simulink model "ass2_test_additions"  (R2022b)
settings: Solver=FixedStepAuto  StartTime=0.0  StopTime=10.0  FixedStep=1e-3  RelTol=1e-3  EnableMultiTasking=on
undefined symbols (not defined in the file): a, b, c, D0, D1, D10, D11, D12, D13, D2, D3, D4, D5, D6, D7, D8, D9, PTA0, PTA1, PTA2, PTB23, PTB9, PTC16, PTC17, PTC2, PTC3, PTC4, PTD0, PTD1, PTD2, PTD3
libraries: frdmk64flib x18, simulink x2, dspstat3 x1, hdlsllib x1
settings Model: ExtModeTrigDuration=5  Creator=hinda  LastModifiedBy=Venka
settings SolverCC: AlgebraicLoopSolver=TrustRegion
settings OptimizationCC: EnhancedBackFolding=on  PassReuseOutputArgsAs=Individual arguments  ZeroExternalMemoryAtStartup=off  ZeroInternalMemoryAtStartup=off  MaxStackSize=64  OptimizeBlockOrder=speed  DifferentSizesBufferReuse=on  OptimizationCustomize=off  EfficientTunableParamExpr=on
settings DebuggingCC: ParameterTunabilityLossMsg=error  UnconnectedInputMsg=warning  UnconnectedOutputMsg=warning  UnconnectedLineMsg=warning  SFMachineParentedDataDiag=warning
settings HardwareCC: ProdBitPerPointer=32  ProdBitPerSizeT=32  ProdBitPerPtrDiffT=32  ProdLargestAtomicInteger=Long  ProdLargestAtomicFloat=Double  ProdWordSize=32  ProdHWDeviceType=ARM Compatible->ARM Cortex
settings ModelReferenceCC: EnableRefExpFcnMdlSchedulingChecks=on
settings SFSimCC: MATLABDynamicMemAlloc=off
settings RTWCC: Description=Embedded Coder  SystemTargetFile=ert.tlc  HardwareBoard=NXP FRDM-K64F  TLCOptions="-aInlineSetEventsForThisBaseRateFcn=TLC_FALSE -aSuppressMultiTaskScheduler=TLC_FALSE  -aRateBasedStepFcn=0"  TemplateMakefile=ert_default_tmf  Toolchain=GNU Tools for ARM Embedded Processors
settings CodeAppCC: ForceParamTrailComments=on  IgnoreCustomStorageClasses=off  OperatorAnnotations=on  SimulinkDataObjDesc=on  SFDataObjDesc=on  InsertBlockDesc=on

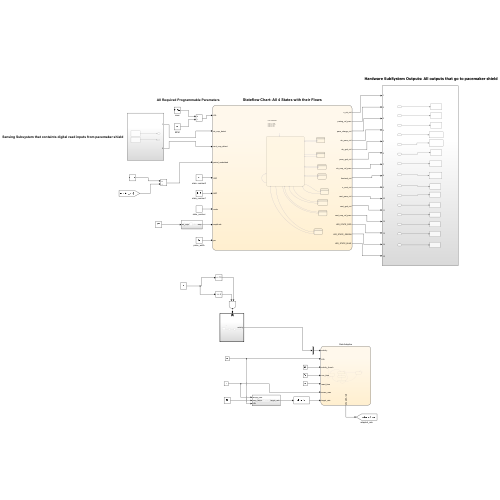
[thumbnail: Simulink's stored preview of the top-level diagram]
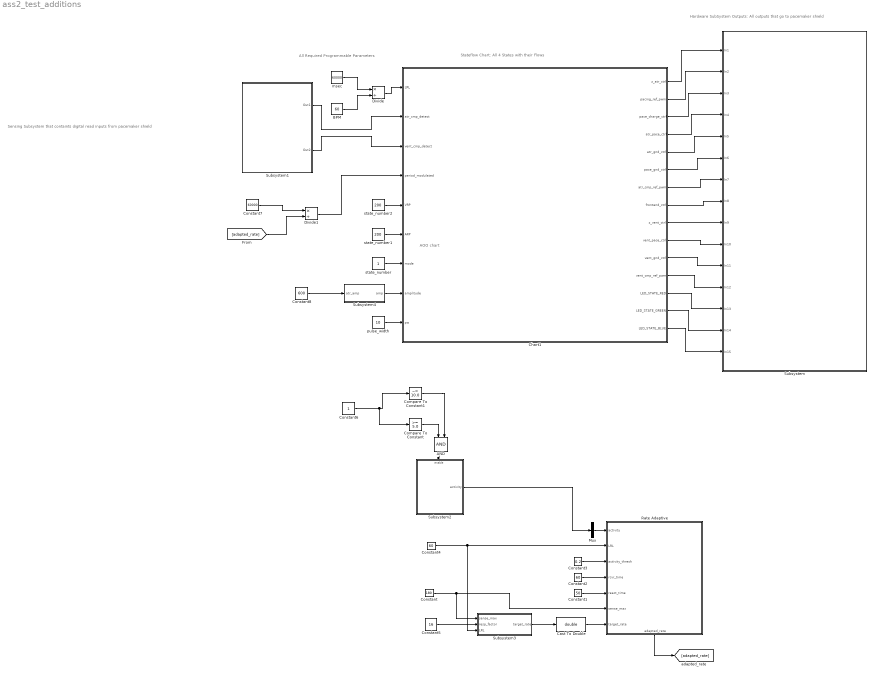
== system ass2_test_additions ==
  note: Sensing Subsystem that containts digital read inputs from pacemaker shield
  note: All Required Programmable Parameters
  note: Hardware SubSystem Outputs: All outputs that go to pacemaker shield
  note: AOO chart
  note: Stateflow Chart: All 4 States with their Flows
  AND : Logic  IconShape=distinctive  AllPortsSameDT=off  OutDataTypeStr=boolean
  BPM : Constant  Value=60
  Cast To Double : DataTypeConversion  OutDataTypeStr=double  SaturateOnIntegerOverflow=off  RndMeth=Floor
  Chart1 : Stateflow chart  TreatAsAtomicUnit=on
      settings: PortSchema="{\"entries\":[{\"content\":{\"sides\":[{\"content\":{\"connectorIds\":[\"In1\",\"In2\",\"In6\",\"In7\",\"In8\",\"In9\",\"In3\",\"In4\",\"In5\"]},\"type\":\"ConnectorPlacement.EquallySpacedRectSide\",\"uuid\":\"9ebc7a7a-d83d-48fa-a96d-77ac692b9900\"},{\"content\":{\"connectorIds\":[\"Out1\",\"Out2\",\"Out3\",\"Out4\",\"Out5\",\"Out6\",\"Out7\",\"Out8\",\"Out9\",\"Out10\",\"Out11\",\"Out12\",\"Out13\",\"Out14\",\"Out15\"],\"side\":\"RIGHT\"},\"type\":\"ConnectorPlacement.EquallySpacedRectSide\",\"uuid\":\"b238fc19-89ba-47ab-b52b-92ee760fd465\"},{\"content\":{\"connectorIds\":[],\"side\":\"TOP\"},\"type\":\"ConnectorPlacement.EquallySpacedRectSide\",\"uuid\":\"260cfadc-f762-444a-84c6-2a5806da8ce4\"}]},\"type\":\"ConnectorPlacement.EquallySpacedConnector\",\"uuid\":\"de40cf96-4d97-4a60-8c1b-853002d7031e\"}],\"packageUris\":[\"http://schema.mathworks.com/mf0/Connector/19700101\"],\"version\":\"1.0\"}"
  Compare To Constant : simulink/Logic and Bit Operations/Compare To Constant  relop=>=  const=5.0  OutDataTypeStr=boolean
  Compare To Constant1 : simulink/Logic and Bit Operations/Compare To Constant  relop=~=  const=10.0  OutDataTypeStr=boolean
  Constant : Constant  Value=180
  Constant1 : Constant  Value=50
  Constant2 : Constant  Value=60
  Constant3 : Constant  Value=0.2
  Constant4 : Constant  Value=60
  Constant5 : Constant  Value=16
  Constant6 : Constant
  Constant7 : Constant  Value=60000
  Constant8 : Constant  Value=600
  Divide : Product  Inputs=*/
  Divide1 : Product  Inputs=*/
  Mux : Mux  Inputs=1
  Rate Adaptive : Stateflow chart  TreatAsAtomicUnit=on
      settings: PortSchema="{\"entries\":[{\"content\":{\"sides\":[{\"content\":{\"connectorIds\":[\"In1\",\"In2\",\"In3\",\"In4\",\"In5\",\"In6\",\"In7\"]},\"type\":\"ConnectorPlacement.EquallySpacedRectSide\",\"uuid\":\"9bfc4146-289d-4395-9573-484b585283b2\"},{\"content\":{\"connectorIds\":[],\"side\":\"RIGHT\"},\"type\":\"ConnectorPlacement.EquallySpacedRectSide\",\"uuid\":\"dae88dc0-efd3-40ed-bd4b-769c24bc4780\"},{\"content\":{\"connectorIds\":[],\"side\":\"TOP\"},\"type\":\"ConnectorPlacement.EquallySpacedRectSide\",\"uuid\":\"b25965ae-4dae-487f-9d9a-0db6d0400c2a\"},{\"content\":{\"connectorIds\":[\"Out1\"],\"side\":\"BOTTOM\"},\"type\":\"ConnectorPlacement.EquallySpacedRectSide\",\"uuid\":\"eb6b3b73-f824-43c6-a49f-c0d69805790b\"}]},\"type\":\"ConnectorPlacement.EquallySpacedConnector\",\"uuid\":\"997eca09-973f-4fce-b3a0-baa9e99f563a\"}],\"packageUris\":[\"http://schema.mathworks.com/mf0/Connector/19700101\"],\"version\":\"1.0\"}"
  Subsystem : Subsystem
  Subsystem1 : Subsystem
  Subsystem2 : Subsystem
  Subsystem3 : Subsystem
  Subsystem4 : Subsystem
  msec : Constant  Value=60000
  pulse_width : Constant  Value=10
  state_number : Constant
  state_number1 : Constant  Value=200
  state_number2 : Constant  Value=200
  wires:
  Chart1/12(vent_cmp_ref_pwm) -> Subsystem/12(In12)
  BPM/1 -> Divide/2
  Chart1/2(pacing_ref_pwm) -> Subsystem/2(In2)
  Chart1/15(LED_STATE_BLUE) -> Subsystem/15(In15)
  Subsystem1/2(Out2) -> Chart1/6(vent_cmp_detect)
  Divide/1 -> Chart1/1(LRL)
  msec/1 -> Divide/1
  state_number/1 -> Chart1/3(mode)
  Chart1/1(z_atr_ctrl) -> Subsystem/1(In1)
  Chart1/14(LED_STATE_GREEN) -> Subsystem/14(In14)
  Chart1/11(vent_gnd_ctrl) -> Subsystem/11(In11)
  Chart1/9(z_vent_ctrl) -> Subsystem/9(In9)
  Subsystem1/1(Out1) -> Chart1/2(atr_cmp_detect)
  Subsystem4/1(amp) -> Chart1/4(amplitude)
  pulse_width/1 -> Chart1/5(pw)
  Chart1/5(atr_gnd_ctrl) -> Subsystem/5(In5)
  Chart1/3(pace_charge_ctrl) -> Subsystem/3(In3)
  Chart1/7(atr_cmp_ref_pwm) -> Subsystem/7(In7)
  Chart1/6(pace_gnd_ctrl) -> Subsystem/6(In6)
  Chart1/13(LED_STATE_RED) -> Subsystem/13(In13)
  Chart1/4(atr_pace_ctrl) -> Subsystem/4(In4)
  Chart1/10(vent_pace_ctrl) -> Subsystem/10(In10)
  Chart1/8(frontend_ctrl) -> Subsystem/8(In8)
  state_number1/1 -> Chart1/9(ARP)
  state_number2/1 -> Chart1/8(VRP)
  Compare To Constant/1 -> AND/1
  Compare To Constant1/1 -> AND/2
  AND/1 -> Subsystem2/Enable
  Subsystem2/1(activity) -> Mux/1
  Mux/1 -> Rate Adaptive/1(activity)
  Constant4/1 -> Rate Adaptive/2(LRL), Subsystem3/3(LRL)
  Constant2/1 -> Rate Adaptive/4(rcvr_time)
  Constant1/1 -> Rate Adaptive/5(react_time)
  Constant3/1 -> Rate Adaptive/3(activity_thresh)
  Constant5/1 -> Subsystem3/2(resp_factor)
  Cast To Double/1 -> Rate Adaptive/7(target_rate)
  Constant/1 -> Rate Adaptive/6(sense_max), Subsystem3/1(sense_max)
  Subsystem3/1(target_rate) -> Cast To Double/1
  Constant6/1 -> Compare To Constant/1, Compare To Constant1/1
  Rate Adaptive/1(adapted_rate) -> [adapted_rate]
  Constant7/1 -> Divide1/1
  [adapted_rate] -> Divide1/2
  Divide1/1 -> Chart1/7(period_modulated)
  Constant8/1 -> Subsystem4/1(atr_amp)

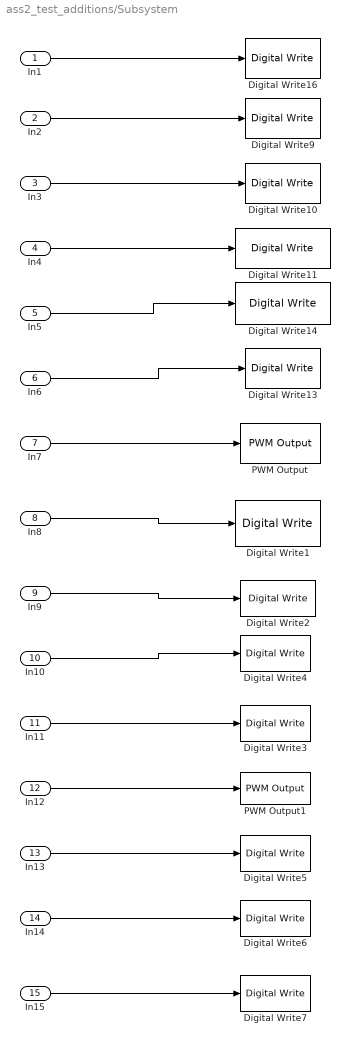
== system ass2_test_additions/Subsystem ==
  In1 : Inport
  In2 : Inport  Port=2
  In3 : Inport  Port=3
  In4 : Inport  Port=4
  In5 : Inport  Port=5
  In6 : Inport  Port=6
  In7 : Inport  Port=7
  In8 : Inport  Port=8
  In9 : Inport  Port=9
  In10 : Inport  Port=10
  In11 : Inport  Port=11
  In12 : Inport  Port=12
  In13 : Inport  Port=13
  In14 : Inport  Port=14
  In15 : Inport  Port=15
  Digital Write1 : frdmk64flib/Digital Write  Whichpin=PTD1 (D13)
  Digital Write10 : frdmk64flib/Digital Write  Whichpin=PTB9 (D2)
  Digital Write11 : frdmk64flib/Digital Write  Whichpin=PTA0 (D8)
  Digital Write13 : frdmk64flib/Digital Write  Whichpin=PTD0 (D10)
  Digital Write14 : frdmk64flib/Digital Write  Whichpin=PTD2 (D11)
  Digital Write16 : frdmk64flib/Digital Write  Whichpin=PTB23 (D4)
  Digital Write2 : frdmk64flib/Digital Write  Whichpin=PTC3 (D7)
  Digital Write3 : frdmk64flib/Digital Write  Whichpin=PTD3 (D12)
  Digital Write4 : frdmk64flib/Digital Write  Whichpin=PTC4 (D9)
  Digital Write5 : frdmk64flib/Digital Write  Whichpin=RED_LED
  Digital Write6 : frdmk64flib/Digital Write  Whichpin=GREEN_LED
  Digital Write7 : frdmk64flib/Digital Write  Whichpin=BLUE_LED
  Digital Write9 : frdmk64flib/Digital Write  Whichpin=PTA2 (D5)
  PWM Output : frdmk64flib/PWM Output  Whichpin=PTC2 (D6)  InitialFrequency=2000  InitialDutyCycle=0
  PWM Output1 : frdmk64flib/PWM Output  Whichpin=PTA1 (D3)  InitialFrequency=2000  InitialDutyCycle=0
  wires:
  In1/1 -> Digital Write16/1
  In2/1 -> Digital Write9/1
  In3/1 -> Digital Write10/1
  In4/1 -> Digital Write11/1
  In5/1 -> Digital Write14/1
  In6/1 -> Digital Write13/1
  In7/1 -> PWM Output/1
  In8/1 -> Digital Write1/1
  In9/1 -> Digital Write2/1
  In10/1 -> Digital Write4/1
  In11/1 -> Digital Write3/1
  In12/1 -> PWM Output1/1
  In13/1 -> Digital Write5/1
  In14/1 -> Digital Write6/1
  In15/1 -> Digital Write7/1

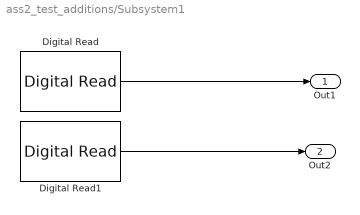
== system ass2_test_additions/Subsystem1 ==
  Digital Read : frdmk64flib/Digital Read  Whichpin=PTC16 (D0)  SampleTime=-1
  Digital Read1 : frdmk64flib/Digital Read  Whichpin=PTC17 (D1)  SampleTime=-1
  Out1 : Outport
  Out2 : Outport  Port=2
  wires:
  Digital Read/1 -> Out1/1
  Digital Read1/1 -> Out2/1

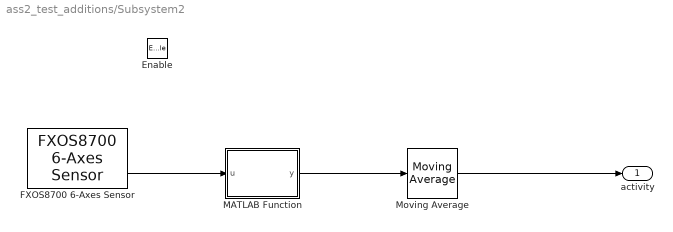
== system ass2_test_additions/Subsystem2 ==
  Enable : EnablePort
  FXOS8700 6-Axes Sensor : frdmk64flib/FXOS8700 6-Axes Sensor  Activesensor=Accelerometer and Magnetometer  ODR=800Hz  HybridODR=400Hz  Accelfullrange=-4g to +4g  SampleTime=-1
  MATLAB Function : MATLAB Function  TreatAsAtomicUnit=on
  Moving Average : dspstat3/Moving Average  Method=Sliding window  ForgettingFactorPort=off  SpecifyWindowLength=on  WindowLength=4  OverlapLength=3  AllowArbitraryInputLength=off  ForgettingFactor=0.9  SimulateUsing=Code generation
  activity : Outport
  wires:
  FXOS8700 6-Axes Sensor/2 -> MATLAB Function/1(u)
  MATLAB Function/1(y) -> Moving Average/1
  Moving Average/1 -> activity/1

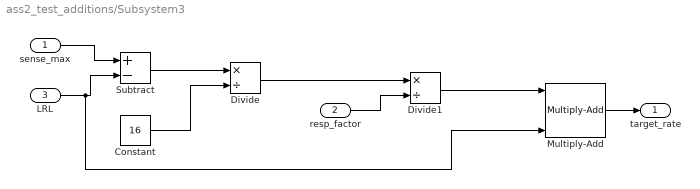
== system ass2_test_additions/Subsystem3 ==
  sense_max : Inport
  resp_factor : Inport  Port=2
  LRL : Inport  Port=3
  Constant : Constant  Value=16
  Divide : Product  Inputs=*/
  Divide1 : Product  Inputs=*/
  Multiply-Add : hdlsllib/HDL Operations/Multiply-Add  Function=c+(a.*b)  datatype=Inherit: Inherit via internal rule  DoSatur=off  FMA=off
  Subtract : Sum  Inputs=+-
  target_rate : Outport
  wires:
  sense_max/1 -> Subtract/1
  LRL/1 -> Multiply-Add/3, Subtract/2
  Subtract/1 -> Divide/1
  Constant/1 -> Divide/2
  Divide/1 -> Divide1/1
  resp_factor/1 -> Divide1/2
  Divide1/1 -> Multiply-Add/1
  Multiply-Add/1 -> target_rate/1

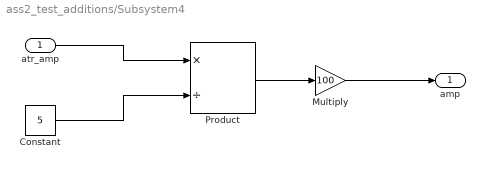
== system ass2_test_additions/Subsystem4 ==
  atr_amp : Inport
  Constant : Constant  Value=5
  Multiply : Gain  Gain=100
  Product : Product  Inputs=*/
  amp : Outport
  wires:
  Product/1 -> Multiply/1
  atr_amp/1 -> Product/1
  Constant/1 -> Product/2
  Multiply/1 -> amp/1

== stateflow chart ass2_test_additions/Chart1 ==
  note: LIST OF MODES
      |
      | mode 1 = AOO
      | mode 2 = VOO
      | mode 3 = AAI
      | mode 4 = VVI
  note: Initializes all variables that will be used for charging and pacing modes
  note: start_here
  state INIT
    entry:
    z_vent_ctrl = 0;
    z_atr_ctrl = 0;
    pace_charge_ctrl=0;
    vent_pace_ctrl = 0;
    atr_pace_ctrl = 0;
    atr_gnd_ctrl = 0;
    vent_gnd_ctrl = 0;
    pace_gnd_ctrl = 0;
    frontend_ctrl = 1;
    atr_cmp_ref_pwm = 80;
    vent_cmp_ref_pwm = 80;
    %LRL is what tells you when to send in a pulse if
    %incoming rate is lower than LRL
  state AOO
    state pacing
      entry:
      %charging C21
      %discharging C22
      atr_gnd_ctrl = 0;
      atr_pace_ctrl = 1;
      z_atr_ctrl = 0;
      pace_charge_ctrl = 0;
      pace_gnd_ctrl = 1;
      atr_gnd_ctrl = 0;
      pacing_ref_pwm = amplitude;
    state charging
      entry:
      %charging C22
      %discharging C21
      atr_pace_ctrl = 0; %do not want c22 to discharge
      pacing_ref_pwm = amplitude; %send in signal
      pace_charge_ctrl = 1;
      pace_gnd_ctrl = 0; %discharges C21
      atr_gnd_ctrl = 1; %1 when discharging through atrium
      atr_cmp_ref_pwm = 80; %send in threshold signal, if heart is less then we will send signal
      %average threshold amplitude is 80
      z_atr_ctrl = 0; %connects impedance circuit to atrium ring electrode output is at z_signal pin
    AOO.charging -> pacing [order 1] : [after(LRL - pw, msec)]
    pacing -> AOO.charging : [after(pw, msec)]
  state VOO
    state charging1
      entry:
      %charging C22
      %discharging C21
      vent_pace_ctrl = 0; %do not want c22 to discharge
      pacing_ref_pwm = amplitude; %send in signal
      pace_charge_ctrl = 1;
      pace_gnd_ctrl = 0; %discharges C21
      vent_gnd_ctrl = 1; %1 when discharging through VENT
      vent_cmp_ref_pwm = 80; %send in threshold signal, if heart is less then we will send signal
      %average threshold amplitude is 80
      z_vent_ctrl = 0; %connects impedance circuit to atrium ring electrode output is at z_signal pin
      LED_STATE_RED=0;
      LED_STATE_GREEN=1;
    state pacing1
      entry:
      %charging C21
      %discharging C22
      vent_gnd_ctrl = 0;
      vent_pace_ctrl = 1;
      z_vent_ctrl = 0;
      pace_charge_ctrl = 0;
      pace_gnd_ctrl = 1;
      vent_gnd_ctrl = 0;
      pacing_ref_pwm = amplitude;
      LED_STATE_RED=1;
      LED_STATE_GREEN=0;
    charging1 -> pacing1 [order 1] : [after(LRL - pw, msec)]
    pacing1 -> charging1 : [after(pw, msec)]
  state AAI
    state charging2
      entry:
      %CHARGING
      %charging C22
      %discharging C21
      atr_pace_ctrl = 0; %do not want c22 to discharge
      pacing_ref_pwm = amplitude; %send in signal
      pace_charge_ctrl = 1;
      pace_gnd_ctrl = 0; %discharges C21
      atr_gnd_ctrl = 1; %1 when discharging through atr
      %average threshold amplitude is 80
      z_atr_ctrl = 0; %connects impedance circuit to atrium ring electrode output is at z_signal pin
      %SENSING
      frontend_ctrl = 1;
      atr_cmp_ref_pwm = 80; %send in threshold signal, if heart is less then we will send signal
      LED_STATE_RED = 1;
      LED_STATE_BLUE = 0;
    state pacing2
      entry:
      %charging C21
      %discharging C22
      atr_gnd_ctrl = 0;
      atr_pace_ctrl = 1;
      z_atr_ctrl = 0;
      pace_charge_ctrl = 0;
      pace_gnd_ctrl = 1;
      pacing_ref_pwm = amplitude;
      frontend_ctrl = 0;
      LED_STATE_RED = 0;
      LED_STATE_BLUE = 1;
    (junction 250) -> charging2 [order 1] : [atr_cmp_detect == 1]
    charging2 -> (junction 250) [order 1]
    (junction 250) -> pacing2 [order 2] : after(LRL-pw, msec)[atr_cmp_detect==0]
    pacing2 -> charging2 : [after(pw, msec)]
  state VVI
    state charging3
      entry:
      %CHARGING
      %charging C22
      %discharging C21
      vent_pace_ctrl = 0; %do not want c22 to discharge
      pacing_ref_pwm = amplitude; %send in signal
      pace_charge_ctrl = 1;
      pace_gnd_ctrl = 0; %discharges C21
      vent_gnd_ctrl = 1; %1 when discharging through vent
      %average threshold amplitude is 80
      z_vent_ctrl = 0; %connects impedance circuit to vent ring electrode output is at z_signal pin
      %SENSING
      frontend_ctrl = 1;
      vent_cmp_ref_pwm = 80; %send in threshold signal, if heart is less then we will send signal
      LED_STATE_RED=1;
      LED_STATE_GREEN=0;
    state pacing3
      entry:
      %charging C21
      %discharging C22
      vent_gnd_ctrl = 0;
      vent_pace_ctrl = 1;
      z_vent_ctrl = 0;
      pace_charge_ctrl = 0;
      pace_gnd_ctrl = 1;
      pacing_ref_pwm = amplitude;
      frontend_ctrl = 0;
      LED_STATE_RED=0;
      LED_STATE_GREEN=1;
    (junction 263) -> charging3 [order 1] : [vent_cmp_detect == 1]
    charging3 -> (junction 263) [order 1]
    (junction 263) -> pacing3 [order 2] : after(LRL-pw, msec)[vent_cmp_detect==0]
    pacing3 -> charging3 : [after(pw, msec)]
  state AOOR
    state charging5
      entry:
      %charging C22
      %discharging C21
      atr_pace_ctrl = 0; %do not want c22 to discharge
      pacing_ref_pwm = amplitude; %send in signal
      pace_charge_ctrl = 1;
      pace_gnd_ctrl = 0; %discharges C21
      atr_gnd_ctrl = 1; %1 when discharging through atrium
      atr_cmp_ref_pwm = 80; %send in threshold signal, if heart is less then we will send signal
      %average threshold amplitude is 80
      z_atr_ctrl = 0; %connects impedance circuit to atrium ring electrode output is at z_signal pin
    state pacing4
      entry:
      %charging C21
      %discharging C22
      atr_gnd_ctrl = 0;
      atr_pace_ctrl = 1;
      z_atr_ctrl = 0;
      pace_charge_ctrl = 0;
      pace_gnd_ctrl = 1;
      atr_gnd_ctrl = 0;
      pacing_ref_pwm = amplitude;
    charging5 -> pacing4 [order 1] : [after(period_modulated - pw, msec)]
    pacing4 -> charging5 : [after(pw, msec)]
  state VOOR
    state charging4
      entry:
      %charging C22
      %discharging C21
      vent_pace_ctrl = 0; %do not want c22 to discharge
      pacing_ref_pwm = amplitude; %send in signal
      pace_charge_ctrl = 1;
      pace_gnd_ctrl = 0; %discharges C21
      vent_gnd_ctrl = 1; %1 when discharging through VENT
      vent_cmp_ref_pwm = 80; %send in threshold signal, if heart is less then we will send signal
      %average threshold amplitude is 80
      z_vent_ctrl = 0; %connects impedance circuit to atrium ring electrode output is at z_signal pin
      LED_STATE_RED=0;
      LED_STATE_GREEN=1;
    state pacing7
      entry:
      %charging C21
      %discharging C22
      vent_gnd_ctrl = 0;
      vent_pace_ctrl = 1;
      z_vent_ctrl = 0;
      pace_charge_ctrl = 0;
      pace_gnd_ctrl = 1;
      vent_gnd_ctrl = 0;
      pacing_ref_pwm = amplitude;
      LED_STATE_RED=1;
      LED_STATE_GREEN=0;
    charging4 -> pacing7 [order 1] : [after(period_modulated - pw, msec)]
    pacing7 -> charging4 : [after(pw, msec)]
  state AAIR
    state charging
      during:
      %CHARGING
      %charging C22
      %discharging C21
      pacing_ref_pwm = amplitude; %send in signal
      atr_pace_ctrl = 0;
      vent_pace_ctrl = 0;
      pace_charge_ctrl = 1;
      pace_gnd_ctrl = 1;
      vent_pace_ctrl = 0;
      z_atr_ctrl = 0;
      z_vent_ctrl = 0;
      atr_pace_ctrl = 0;
      atr_gnd_ctrl = 1;
      vent_gnd_ctrl = 0;
    state discharging
      during:
      pace_charge_ctrl = 0;
      pace_gnd_ctrl = 1;
      atr_pace_ctrl = 1;
      atr_gnd_ctrl = 0;
      z_atr_ctrl = 0;
      z_vent_ctrl = 0;
      vent_gnd_ctrl = 0;
      vent_pace_ctrl = 0;
    state choosing
      during:
      pace_gnd_ctrl = 1;
      vent_pace_ctrl  = 0;
      z_atr_ctrl  = 0;
      z_vent_ctrl  = 0;
      atr_pace_ctrl  = 0;
      atr_gnd_ctrl  = 1;
      vent_gnd_ctrl = 0;
      atr_pace_ctrl  = 0;
      vent_pace_ctrl  = 0;
      pacing_ref_pwm = amplitude;
      pace_charge_ctrl = 1;
      frontend_ctrl = 1;
    AAIR.charging -> AAIR.discharging [order 1] : after(period_modulated - pw - ARP, msec)
    AAIR.charging -> (junction 320) [order 3] : [atr_cmp_detect == 1]
    (junction 320) -> AAIR.choosing : after(LRL, msec)
    AAIR.discharging -> AAIR.choosing : after(pw, msec)
    AAIR.choosing -> AAIR.charging : after(ARP, msec)
  state VVIR
    state charging
      during:
      %CHARGING
      %charging C22
      %discharging C21
      pacing_ref_pwm = amplitude; %send in signal
      atr_pace_ctrl = 0;
      vent_pace_ctrl = 0;
      pace_charge_ctrl = 1;
      pace_gnd_ctrl = 1;
      vent_pace_ctrl = 0;
      z_atr_ctrl = 0;
      z_vent_ctrl = 0;
      atr_pace_ctrl = 0;
      atr_gnd_ctrl = 0;
      vent_gnd_ctrl = 1;
    state discharging
      during:
      pace_charge_ctrl = 0;
      pace_gnd_ctrl = 1;
      atr_pace_ctrl = 0;
      atr_gnd_ctrl = 0;
      z_atr_ctrl = 0;
      z_vent_ctrl = 0;
      vent_gnd_ctrl = 0;
      vent_pace_ctrl = 1;
    state choosing
      during:
      pace_gnd_ctrl = 1;
      vent_pace_ctrl  = 0;
      z_atr_ctrl  = 0;
      z_vent_ctrl  = 0;
      atr_pace_ctrl  = 0;
      atr_gnd_ctrl  = 0;
      vent_gnd_ctrl = 1;
      atr_pace_ctrl  = 0;
      vent_pace_ctrl  = 0;
      pacing_ref_pwm = amplitude;
      pace_charge_ctrl = 1;
    VVIR.charging -> VVIR.discharging [order 2] : after(period_modulated - pw - VRP, msec)
    VVIR.charging -> (junction 317) [order 3] : [vent_cmp_detect == 1]
    (junction 317) -> VVIR.choosing : after(LRL, msec)
    VVIR.discharging -> VVIR.choosing : after(pw, msec)
    VVIR.choosing -> VVIR.charging : after(VRP, msec)
  AAIR.charging -> INIT [order 2] : [mode ~=7]
  charging5 -> INIT [order 2] : [mode ~= 5]
  charging3 -> INIT [order 2] : [mode ~=4]
  charging4 -> INIT [order 2] : [mode ~= 6]
  AOO.charging -> INIT [order 2] : [mode ~= 1]
  charging1 -> INIT [order 2] : [mode ~= 2]
  VVIR.charging -> INIT [order 1] : [mode ~= 8]
  INIT -> AAIR.charging [order 9] : [mode ==7]
  charging2 -> INIT [order 2] : [mode ~=3]
  INIT -> AOO.charging [order 2] : [mode ==1]
  (default) -> INIT
  INIT -> charging1 [order 3] : [mode == 2]
  INIT -> charging5 [order 7] : [mode ==5]
  INIT -> charging2 [order 6] : [mode ==3]
  INIT -> INIT [order 8] : [mode ~= 1 | mode ~= 2 | mode ~= 3 | mode ~= 4 | mode~= 5| mode ~= 6| mode~=7| mode~=8]
  INIT -> charging3 [order 4] : [mode == 4]
  INIT -> charging4 [order 5] : [mode == 6]
  INIT -> VVIR.charging [order 1] : [mode == 8]
  data: LRL input; z_atr_ctrl output; pacing_ref_pwm output; pace_charge_ctrl output; atr_pace_ctrl output; atr_gnd_ctrl output; pace_gnd_ctrl output; atr_cmp_ref_pwm output; atr_cmp_detect input; frontend_ctrl output; mode input; amplitude input; pw input; vent_cmp_detect input; z_vent_ctrl output; vent_pace_ctrl output; vent_gnd_ctrl output; vent_cmp_ref_pwm output; LED_STATE_RED output; LED_STATE_GREEN output; LED_STATE_BLUE output; period_modulated input; VRP input; ARP input

== matlab function ass2_test_additions/Subsystem2/MATLAB Function ==
  data: u input; y output
function y = fcn(u)

y = sqrt(u(1)^2+u(2)^2+u(3)^2);

== stateflow chart ass2_test_additions/Rate Adaptive ==
  state Start2
    entry:
    adapted_rate = adapted_rate + step_up;
  state Start5
    entry:
    adapted_rate = target_rate
  state Start
    entry:
    adapted_rate = LRL;
  state Start3
    entry:
    adapted_rate = adapted_rate - step_up;
  state Start4
    entry:
    adapted_rate = adapted_rate - step_down;
  (default) -> Start : {step_up = ceil((sense_max - LRL) / react_time),
      | step_down = ceil((sense_max - LRL)  / rcvr_time)}
  Start -> Start2 [order 2] : [activity >= activity_thresh]
  Start5 -> Start5 [order 1] : [activity > activity_thresh]
  Start2 -> Start2 [order 1] : after(1000,msec)[adapted_rate <= target_rate]
  Start2 -> Start5 [order 3] : [adapted_rate >= target_rate]
  Start2 -> Start4 [order 4] : [activity >= activity_thresh]
  Start2 -> Start3 [order 2] : [activity<activity_thresh]
  Start3 -> Start2 [order 1] : [activity >= activity_thresh]
  Start5 -> Start4 [order 2] : [activity < activity_thresh]
  Start -> Start [order 1] : [activity < activity_thresh]
  Start4 -> Start [order 2] : [adapted_rate <= LRL]
  Start3 -> Start4 [order 2] : after(1000,msec)
  Start4 -> Start4 [order 1] : after(1000, msec)[adapted_rate >= LRL]
  data: activity input; adapted_rate output; LRL input; step_up local; step_down local; activity_thresh input; rcvr_time input; react_time input; sense_max input; target_rate input
